simulink model "hw_control_adapt_PI_EKF"  (R2021b)
settings: Solver=ode1  StartTime=0.0  StopTime=100  FixedStep=0.01  RelTol=1e-3  EnableMultiTasking=on
libraries: arduinolib x2, arduinosensorlib x1
settings Model: PacingRate=3  ExtModeTrigDuration=2  Creator=ONLY-GOD  LastModifiedBy=ASUS
settings SolverCC: AlgebraicLoopSolver=TrustRegion
settings OptimizationCC: EnhancedBackFolding=on  PassReuseOutputArgsAs=Individual arguments  ZeroExternalMemoryAtStartup=off  ZeroInternalMemoryAtStartup=off  MaxStackSize=64  OptimizeBlockOrder=speed  DifferentSizesBufferReuse=on  OptimizationCustomize=off  EfficientTunableParamExpr=on
settings DebuggingCC: ParameterTunabilityLossMsg=error  SFMachineParentedDataDiag=warning
settings HardwareCC: ProdBitPerInt=16  ProdBitPerPointer=16  ProdBitPerSizeT=16  ProdBitPerPtrDiffT=16  ProdLargestAtomicFloat=None  ProdWordSize=8  ProdHWDeviceType=Atmel->AVR
settings SFSimCC: MATLABDynamicMemAlloc=off
settings RTWCC: Description=Embedded Coder  SystemTargetFile=ert.tlc  HardwareBoard=Arduino Mega 2560  TemplateMakefile=ert_default_tmf  Toolchain=Arduino AVR  BuildConfiguration=Faster Runs
settings CodeAppCC: ForceParamTrailComments=on  IgnoreCustomStorageClasses=off  OperatorAnnotations=on  SimulinkDataObjDesc=on  SFDataObjDesc=on  InsertBlockDesc=on
settings ERTTargetCC: SupportContinuousTime=on  SupportVariableSizeSignals=on  ExtModeTransport=3  ExtModeStaticAlloc=on  ExtModeStaticAllocSize=2048  ExtModeMexFile=ext_xcp  ExtModeIntrfLevel=Level2 - Open

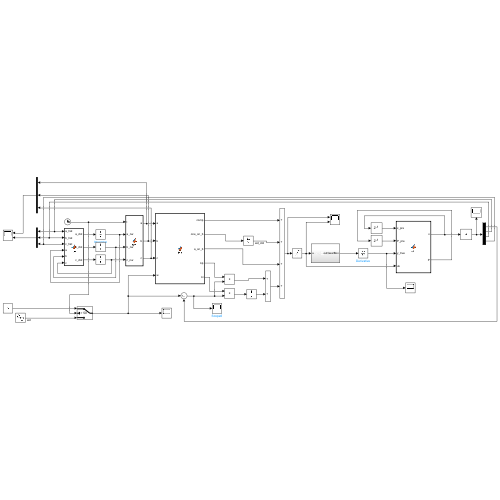
[thumbnail: Simulink's stored preview of the top-level diagram]
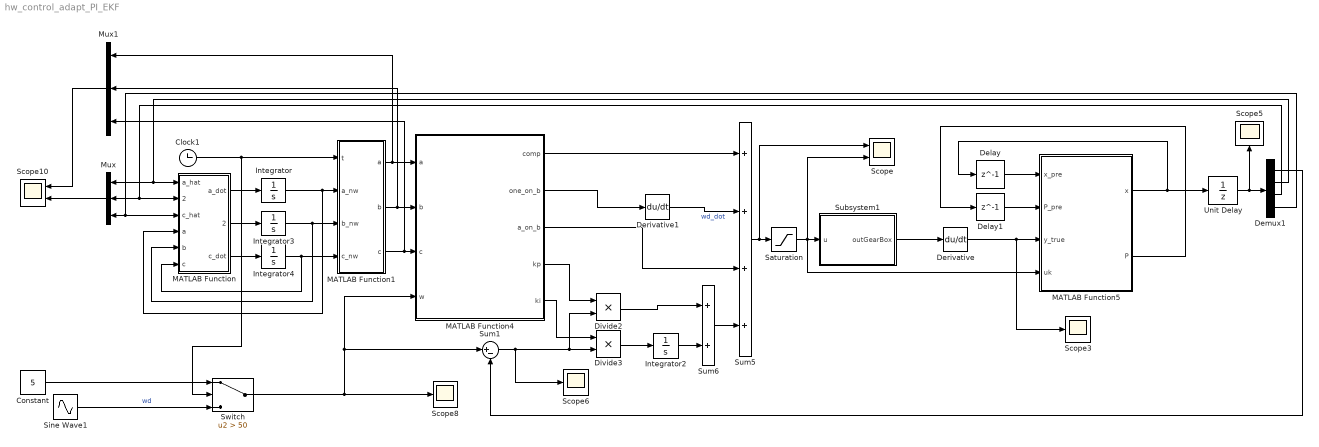
== system hw_control_adapt_PI_EKF ==
  Clock1 : Clock
  Constant : Constant  Value=5
  Delay : Delay  DelayLength=1  InitialCondition=[0;0;0;0]
  Delay1 : Delay  DelayLength=1  InitialCondition=1e0*diag([10,1,30,10])
  Demux1 : Demux
  Derivative : Derivative
  Derivative1 : Derivative
  Divide2 : Product  Inputs=**
  Divide3 : Product  Inputs=**
  Integrator : Integrator  InitialCondition=24.4300
  Integrator2 : Integrator
  Integrator3 : Integrator  InitialCondition=40.3400
  Integrator4 : Integrator  InitialCondition=18.3700
  MATLAB Function : MATLAB Function  TreatAsAtomicUnit=on
  MATLAB Function1 : MATLAB Function  TreatAsAtomicUnit=on
  MATLAB Function4 : MATLAB Function  TreatAsAtomicUnit=on
  MATLAB Function5 : MATLAB Function  TreatAsAtomicUnit=on
  Mux : Mux  Inputs=3
  Mux1 : Mux  Inputs=3
  Saturation : Saturate  UpperLimit=23  LowerLimit=-23
  Scope : Scope  NumInputPorts=2
  Scope10 : Scope  NumInputPorts=2
  Scope{3,5..6,8} (4 alike) : Scope
  Sine Wave1 : Sin  Amplitude=10  Frequency=2*pi*0.4  SampleTime=0
  Subsystem1 : Subsystem
  Sum1 : Sum  Inputs=|+-
  Sum5 : Sum  Inputs=++++
  Sum6 : Sum
  Switch : Switch  Criteria=u2 > Threshold  Threshold=50
  Unit Delay : UnitDelay  SampleTime=-1  HasFrameUpgradeWarning=on
  wires:
  Subsystem1/1(outGearBox) -> Derivative/1
  MATLAB Function5/2(P) -> Delay1/1
  Delay1/1 -> MATLAB Function5/2(P_pre)
  Delay/1 -> MATLAB Function5/1(x_pre)
  Integrator4/1 -> MATLAB Function1/4(c_nw), MATLAB Function/6(c)
  Divide2/1 -> Sum6/1
  Integrator/1 -> MATLAB Function1/2(a_nw), MATLAB Function/4(a)
  MATLAB Function1/1(a) -> Mux1/1, MATLAB Function4/1(a)
  MATLAB Function/1(a_dot) -> Integrator/1
  Sum6/1 -> Sum5/4
  Integrator3/1 -> MATLAB Function/5(b), MATLAB Function1/3(b_nw)
  MATLAB Function/2(b_dot) -> Integrator3/1
  Demux1/2 -> MATLAB Function/1(a_hat), Mux/1
  Divide3/1 -> Integrator2/1
  Clock1/1 -> Switch/2, MATLAB Function1/1(t)
  Demux1/3 -> MATLAB Function/2(b_hat), Mux/2
  MATLAB Function/3(c_dot) -> Integrator4/1
  MATLAB Function4/1(comp) -> Sum5/1
  MATLAB Function4/3(a_on_b) -> Sum5/3
  Mux/1 -> Scope10/2
  Integrator2/1 -> Sum6/2
  Demux1/4 -> MATLAB Function/3(c_hat), Mux/3
  Mux1/1 -> Scope10/1
  MATLAB Function4/5(ki) -> Divide3/1
  MATLAB Function4/2(one_on_b) -> Derivative1/1
  MATLAB Function4/4(kp) -> Divide2/1
  MATLAB Function1/3(c) -> Mux1/3, MATLAB Function4/3(c)
  Derivative1/1 -> Sum5/2  "wd_dot"
  MATLAB Function1/2(b) -> Mux1/2, MATLAB Function4/2(b)
  Sum1/1 -> Scope6/1, Divide2/2, Divide3/2
  Sum5/1 -> Scope/1, Saturation/1
  Saturation/1 -> MATLAB Function5/4(uk), Scope/2, Subsystem1/1(u)
  Derivative/1 -> Scope3/1, MATLAB Function5/3(y_true)
  MATLAB Function5/1(x) -> Delay/1, Unit Delay/1
  Unit Delay/1 -> Demux1/1, Scope5/1
  Demux1/1 -> Sum1/2
  Sine Wave1/1 -> Switch/3  "wd"
  Switch/1 -> MATLAB Function4/4(w), Sum1/1, Scope8/1
  Constant/1 -> Switch/1

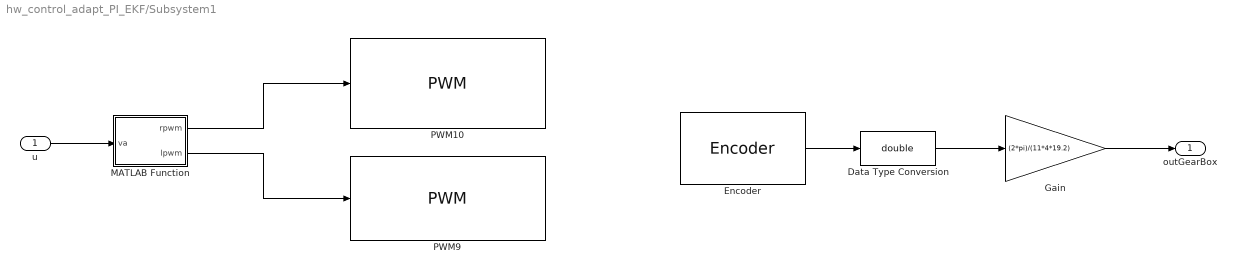
== system hw_control_adapt_PI_EKF/Subsystem1 ==
  u : Inport
  Data Type Conversion : DataTypeConversion  OutDataTypeStr=double
  Encoder : arduinosensorlib/Encoder  InputA=2  InputB=3  Mode=No reset  SampleTime=-1
      settings: SourceProductBaseCode=ARDUINO
  Gain : Gain  Gain=(2*pi)/(11*4*19.2)
  MATLAB Function : MATLAB Function  TreatAsAtomicUnit=on
  PWM10 : arduinolib/PWM  pinNumber=8  frequencyType=Default  desiredFrequency=490.2  achievableFrequency=490.2
  PWM9 : arduinolib/PWM  pinNumber=9  frequencyType=Default  desiredFrequency=490.2  achievableFrequency=490.2
  outGearBox : Outport
  wires:
  Data Type Conversion/1 -> Gain/1
  Gain/1 -> outGearBox/1
  Encoder/1 -> Data Type Conversion/1
  u/1 -> MATLAB Function/1(va)
  MATLAB Function/1(rpwm) -> PWM10/1
  MATLAB Function/2(lpwm) -> PWM9/1

== matlab function hw_control_adapt_PI_EKF/MATLAB Function1 ==
  data: a output; b output; c output; t input; a_nw input; b_nw input; c_nw input
function [a,b,c] = fcn(t,a_nw,b_nw,c_nw)
% a = (2.450e+1 + 2.436e+1)/2;
% b = (4.039e+1 + 4.029e+1)/2;
% c = (1.830e+1 + 1.844e+1)/2;


a = 24.4300;
b = 40.3400;
c = 18.3700;

if t>30
a = a_nw;
b = b_nw;
c = c_nw;
end

== matlab function hw_control_adapt_PI_EKF/MATLAB Function ==
  data: a_hat input; a_dot output; b_hat input; c_hat input; b_dot output; c_dot output; a input; b input; c input
function [a_dot,b_dot,c_dot] = fcn(a_hat,b_hat,c_hat,a,b,c)

lamda = 5;

a_dot = (1/lamda)*(-a+a_hat);
b_dot = (1/lamda)*(-b+b_hat);
c_dot = (1/lamda)*(-c+c_hat);

== matlab function hw_control_adapt_PI_EKF/Subsystem1/MATLAB Function ==
  data: va input; rpwm output; lpwm output
function [rpwm,lpwm] = fcn(va)

pwm = (va/24)*254;

if pwm > 0
    rpwm = pwm;
    lpwm = 0;
elseif pwm<0
    rpwm = 0;
    lpwm = abs(pwm);
else
    rpwm = 0;
    lpwm = 0;
end

== matlab function hw_control_adapt_PI_EKF/MATLAB Function4 ==
  data: comp output; one_on_b output; a input; a_on_b output; b input; c input; w input; kp output; ki output
function [comp,one_on_b,a_on_b,kp,ki] = fcn(a,b,c,w)

a_on_b = (a/b)*w;
one_on_b = (1/b)*w;
comp = (c/b)*sign(w);

wn = 2*pi*6;
zeta = 1;

ki = wn^2/b;
kp = (2*zeta*wn-a)/b;

== matlab function hw_control_adapt_PI_EKF/MATLAB Function5 ==
  settings: updateMethod=DISCRETE
  data: x_pre input; P_pre input; y_true input; x output; uk input; P output
function [x,P] = ekf(x_pre,P_pre,y_true, uk)
Ts = 0.01;

Qc_est  = 1e-4*diag([1,10,100,10]);
Qd_est  = Ts*Qc_est;
R_est   = 0.01;

Ck = [1 0 0 0];
Dk = 0;


% PREDICTION STEP
%Compute prediction at next time step
x = x_pre+Ts*[-x_pre(2)*x_pre(1) + uk*x_pre(3) - x_pre(4)*sign(x_pre(1));
                0;
                0;
                0];

Ak = eye(4)+Ts*[-x_pre(2) -x_pre(1) uk -sign(x_pre(1));
                 0     0    0      0;
                 0     0    0      0;
                 0     0    0      0];
P = Ak*P_pre*Ak'+Qd_est;

% OBSERVATION AND UPDATE
%Comput Kalman Gain and update predicted value
Wk    = P*Ck'/(Ck*P*Ck'+R_est);
y_est = Ck*x+Dk*uk;
dely = y_true-y_est;
Wkdely = Wk*dely;
x = x+Wkdely;
P = P-Wk*Ck*P;
